simulink model "NavV1_0421_2021a"  (R2021a)
settings: Solver=FixedStepAuto  StartTime=0.0  StopTime=589  FixedStep=dt  RelTol=1e-3
values from neighbouring files (symbols this model uses):
  dt = 0.01    [initNavigation.m]
  g0 = 9.798    [initNavigation.m]
  GPSdt = 0.1    [initNavigation.m]
undefined symbols (not defined in the file or in its folder): DiscIntNeverNeededParam, magnitude, param
libraries: simulink x14, simulink_extras x11, sharedtransform x7, dspstat3 x4, aerolibtransform2 x2, dspsolvers x2, aerolibconvert2 x1
(part 2 of 3)

== system NavV1_0421_2021a/State estimation/Translation_estimate/V_Vertical_estimation ==
  note: Vd to Vh
  accel_Vertical_predict : Inport
  Sensor_data : Inport  Port=2
  Vertical_vaild_flag : Inport  Port=3
  Add : Sum
  Add1 : Sum  Inputs=++--
  Bus Selector : BusSelector  OutputSignals=QGC_sensor_reinit,TOF_Data.vH_TOF_m/s_TD,GPS_Data.vd_gps
  Bus Selector1 : BusSelector  OutputSignals=HTOF_vaild,HGPS_vaild
  Constant : Constant  Value=g0  OutDataTypeStr=single
  Delay : Delay  DelayLength=1  InitialConditionSource=Input port  ExternalReset=Level hold
      settings: InputPortMap=u0,r5,p4
  Gain : Gain  Gain=-1
  Gain2 : Gain  Gain=dt  SaturateOnIntegerOverflow=on  OutDataTypeStr=Inherit: Same as input  ParamDataTypeStr=Inherit: Same as input
  Scope : Scope
  Scope1 : Scope  NumInputPorts=3
  VH_correctionbyTOF : Subsystem
  VH_correctionbyTOF1 : Subsystem
  Vh_vertical_eastimate : Outport
  wires:
  Sensor_data/1 -> Bus Selector/1
  Bus Selector/3 -> VH_correctionbyTOF1/2(Vd_gps), Scope1/2, Delay/3  "<vd_gps>"
  Bus Selector/1 -> Delay/2  "<QGC_sensor_reinit>"
  accel_Vertical_predict/1 -> Scope/1, Add/1
  Constant/1 -> Add/2
  Add/1 -> Gain2/1
  Bus Selector/2 -> VH_correctionbyTOF/2(<vH_TOF_m/s_TD>), Scope1/3  "<vH_TOF_m/s_TD>"
  Add1/1 -> Scope1/1, Vh_vertical_eastimate/1, Delay/1, VH_correctionbyTOF/1(VH_k_1), VH_correctionbyTOF1/1(VH_k_1)
  Gain2/1 -> Gain/1
  VH_correctionbyTOF/1(VH_correctionbyTOF) -> Add1/3
  Delay/1 -> Add1/2
  Vertical_vaild_flag/1 -> Bus Selector1/1
  Bus Selector1/1 -> VH_correctionbyTOF/Enable  "<HTOF_vaild>"
  Bus Selector1/2 -> VH_correctionbyTOF1/Enable  "<HGPS_vaild>"
  VH_correctionbyTOF1/1(VH_correctionbyGPS) -> Add1/4
  Gain/1 -> Add1/1

== system NavV1_0421_2021a/State estimation/Translation_estimate/translate to N ==
  RotationData : Inport
  Sensor_data : Inport  Port=2
  Bus Selector2 : BusSelector  OutputSignals=IMU_Data.accl_B_m/s2_LPF
  Bus Selector3 : BusSelector  OutputSignals=DCM_b_n
  Product : Product  Multiplication=Matrix(*)
  Selector : Selector  InputPortWidth=3  IndexOptions=Index vector (dialog)  Indices=[1 2]  OutputSizes=1
  Selector1 : Selector  InputPortWidth=3  IndexOptions=Index vector (dialog)  Indices=[3]  OutputSizes=1
  accel_Horizontal_predict : Outport
  accel_Vertical_predict : Outport  Port=2
  wires:
  RotationData/1 -> Bus Selector3/1
  Bus Selector2/1 -> Product/2  "<accl_B_m/s2_LPF>"
  Bus Selector3/1 -> Product/1  "<DCM_b_n>"
  Sensor_data/1 -> Bus Selector2/1
  Product/1 -> Selector1/1, Selector/1
  Selector/1 -> accel_Horizontal_predict/1
  Selector1/1 -> accel_Vertical_predict/1

== system NavV1_0421_2021a/Sensor_Data_Process/GPS_Data_Process/LLA2NED/Subsystem1 ==
  QGC_sensor_reinit : Inport
  gps_LLA_rad : Inport  Port=2
  Detect Increase : simulink/Logic and Bit Operations/Detect Increase  vinit=0.0  OutDataTypeStr=boolean
  Switch : Switch  Criteria=u2 > Threshold
  Unit Delay : UnitDelay  SampleTime=-1  HasFrameUpgradeWarning=on
  init_gps_LLA0_rad : Outport
  wires:
  Unit Delay/1 -> Switch/3
  gps_LLA_rad/1 -> Switch/1
  Switch/1 -> init_gps_LLA0_rad/1, Unit Delay/1
  Detect Increase/1 -> Switch/2
  QGC_sensor_reinit/1 -> Detect Increase/1

== system NavV1_0421_2021a/State estimation/AHRS/AHRS Complementary filter/Complementary Filter ==
  fbxyz : Inport
  Fly_status : Inport  Port=2
  fb_estimatedValue : Inport  Port=3
  Cross-product : Subsystem
      mask DialogControl Control2 Prompt: Vector A×B
  Gain : Gain  Gain=GPS_accel_kp
  Gain2 : Gain  Gain=noGPS_accel_kp
  Gain3 : Gain  Gain=GPS_accel_ki*dt
  Gain4 : Gain  Gain=noGPS_accel_ki*dt
  Normalized : Subsystem
  Normalized1 : Subsystem
  Sum : Sum  Inputs=|++
  Sum1 : Sum  Inputs=|++
  Switch : Switch  Threshold=2
  w_bias : Outport
  wires:
  Normalized1/1(fb_estimatedValue_Normalized) -> Cross-product/2(vactor_B)
  Normalized/1(fb/g) -> Cross-product/1(vactor_A)
  fbxyz/1 -> Normalized/1(fb)
  fb_estimatedValue/1 -> Normalized1/1(fb_estimatedValue)
  Switch/1 -> w_bias/1
  Fly_status/1 -> Switch/2
  Sum/1 -> Switch/1
  Gain/1 -> Sum/1
  Gain3/1 -> Sum/2
  Cross-product/1(vactor_error_A&B) -> Gain4/1, Gain2/1, Gain3/1, Gain/1
  Gain2/1 -> Sum1/1
  Gain4/1 -> Sum1/2
  Sum1/1 -> Switch/3

== system NavV1_0421_2021a/State estimation/AHRS/AHRS Complementary filter/SmoothModel ==
  bias : Inport
  Demux : Demux  Outputs=3
  Moving Average : dspstat3/Moving Average  Method=Sliding window  ForgettingFactorPort=off  SpecifyWindowLength=on  WindowLength=10  ForgettingFactor=0.9  SimulateUsing=Code generation
  Moving Average1 : dspstat3/Moving Average  Method=Sliding window  ForgettingFactorPort=off  SpecifyWindowLength=on  WindowLength=10  ForgettingFactor=0.9  SimulateUsing=Code generation
  Moving Average2 : dspstat3/Moving Average  Method=Sliding window  ForgettingFactorPort=off  SpecifyWindowLength=on  WindowLength=10  ForgettingFactor=0.9  SimulateUsing=Code generation
  Mux : Mux  Inputs=3
  bias_smooth : Outport
  wires:
  Moving Average/1 -> Mux/1
  Moving Average1/1 -> Mux/2
  Demux/3 -> Moving Average2/1
  Demux/2 -> Moving Average1/1
  Moving Average2/1 -> Mux/3
  Demux/1 -> Moving Average/1
  bias/1 -> Demux/1
  Mux/1 -> bias_smooth/1  "gyro_B_rad/s_LPF"

== system NavV1_0421_2021a/State estimation/AHRS/AHRS Complementary filter/Subsystem6 ==
  m : Inport
  Add : Sum  Inputs=3
  Demux : Demux  Outputs=3
  Display : Display
  Display1 : Display
      settings: Decimation=3
  Divide : Product  Inputs=*/
  Dot Product : DotProduct  InputSameDT=on  OutDataTypeStr=Inherit: Inherit via internal rule
  Dot Product1 : DotProduct  InputSameDT=on  OutDataTypeStr=Inherit: Inherit via internal rule
  Dot Product2 : DotProduct  InputSameDT=on  OutDataTypeStr=Inherit: Inherit via internal rule
  Sqrt : Sqrt  SaturateOnIntegerOverflow=on
  m/|m| : Outport
  wires:
  Demux/2 -> Dot Product1/2, Dot Product1/1
  Demux/3 -> Dot Product2/2, Dot Product2/1
  Divide/1 -> Display1/1, m/|m|/1
  Add/1 -> Sqrt/1
  m/1 -> Demux/1, Divide/1
  Demux/1 -> Dot Product/1, Dot Product/2
  Dot Product1/1 -> Add/2
  Dot Product/1 -> Add/1
  Dot Product2/1 -> Add/3
  Sqrt/1 -> Display/1, Divide/2

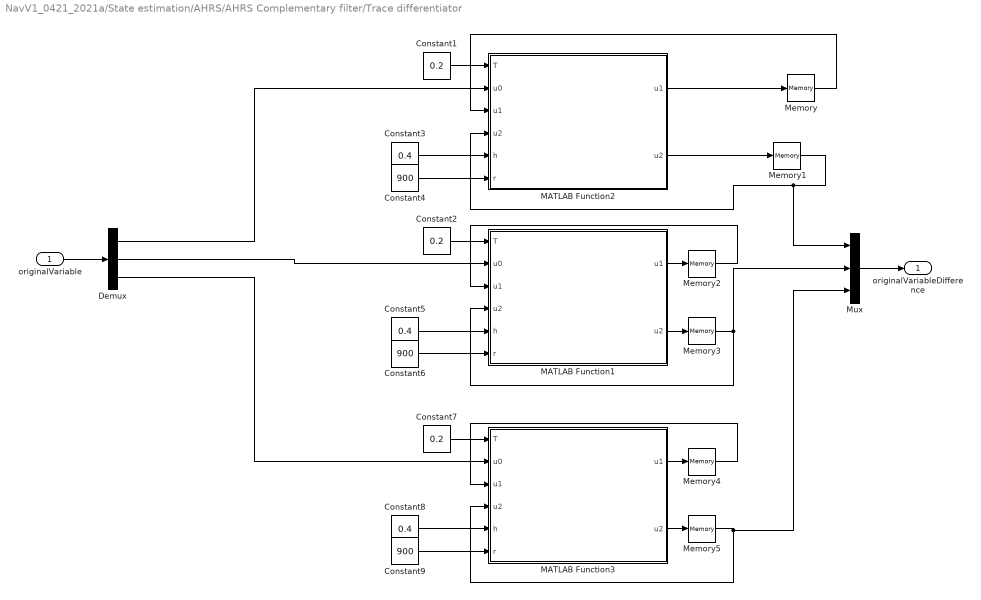
== system NavV1_0421_2021a/State estimation/AHRS/AHRS Complementary filter/Trace differentiator ==
  originalVariable : Inport
  Constant1 : Constant  Value=0.2  OutDataTypeStr=single
  Constant2 : Constant  Value=0.2  OutDataTypeStr=single
  Constant3 : Constant  Value=0.4  OutDataTypeStr=single
  Constant4 : Constant  Value=900  OutDataTypeStr=single
  Constant5 : Constant  Value=0.4  OutDataTypeStr=single
  Constant6 : Constant  Value=900  OutDataTypeStr=single
  Constant7 : Constant  Value=0.2  OutDataTypeStr=single
  Constant8 : Constant  Value=0.4  OutDataTypeStr=single
  Constant9 : Constant  Value=900  OutDataTypeStr=single
  Demux : Demux  Outputs=3
  MATLAB Function1 : MATLAB Function  TreatAsAtomicUnit=on
  MATLAB Function2 : MATLAB Function  TreatAsAtomicUnit=on
  MATLAB Function3 : MATLAB Function  TreatAsAtomicUnit=on
  Memory{,1..5} (6 alike) : Memory  InheritSampleTime=on
  Mux : Mux  Inputs=3
  originalVariableDifference : Outport
  wires:
  Demux/3 -> MATLAB Function3/2(u0)
  Demux/2 -> MATLAB Function1/2(u0)
  Demux/1 -> MATLAB Function2/2(u0)
  originalVariable/1 -> Demux/1
  Mux/1 -> originalVariableDifference/1
  Memory5/1 -> MATLAB Function3/4("u2 "), Mux/3
  Memory4/1 -> MATLAB Function3/3("u1 ")
  MATLAB Function3/2(u2) -> Memory5/1
  Constant8/1 -> MATLAB Function3/5(h)
  Constant7/1 -> MATLAB Function3/1(T)
  Constant9/1 -> MATLAB Function3/6(r)
  MATLAB Function3/1(u1) -> Memory4/1
  MATLAB Function1/1(u1) -> Memory2/1
  Constant6/1 -> MATLAB Function1/6(r)
  Constant2/1 -> MATLAB Function1/1(T)
  Constant5/1 -> MATLAB Function1/5(h)
  MATLAB Function1/2(u2) -> Memory3/1
  Memory2/1 -> MATLAB Function1/3("u1 ")
  Memory3/1 -> Mux/2, MATLAB Function1/4("u2 ")
  Memory1/1 -> MATLAB Function2/4("u2 "), Mux/1
  Memory/1 -> MATLAB Function2/3("u1 ")
  MATLAB Function2/2(u2) -> Memory1/1
  Constant3/1 -> MATLAB Function2/5(h)
  Constant1/1 -> MATLAB Function2/1(T)
  Constant4/1 -> MATLAB Function2/6(r)
  MATLAB Function2/1(u1) -> Memory/1

== system NavV1_0421_2021a/State estimation/AHRS/AHRS Complementary filter/UAV_accelerate_within_gravity_estimate ==
  Fly_status : Inport
  <DCM_b_n> : Inport  Port=2
  accel_GPS_ned : Inport  Port=3
  Add2 : Sum
  Constant : Constant  Value=[0;0;-1]
  Constant1 : Constant  Value=[0;0;0]  OutDataTypeStr=single
  Gain2 : Gain  Gain=g0
  Math Function1 : Math  Operator=transpose  SignedPower=on  SaturateOnIntegerOverflow=on
  Multiport Switch : MultiPortSwitch  Inputs=2  DataPortForDefault=Additional data port
  Product : Product  Multiplication=Matrix(*)  SaturateOnIntegerOverflow=on  OutDataTypeStr=Inherit: Same as first input
  Product1 : Product  Multiplication=Matrix(*)  SaturateOnIntegerOverflow=on  OutDataTypeStr=Inherit: Same as first input
  accelerate_within_gravity_estimate : Outport
  wires:
  <DCM_b_n>/1 -> Math Function1/1
  Math Function1/1 -> Product1/1, Product/1  "DCM_n_b"
  Product1/1 -> Add2/1
  accel_GPS_ned/1 -> Product1/2  "accel_GPS_ned"
  Product/1 -> Gain2/1
  Constant/1 -> Product/2
  Gain2/1 -> Multiport Switch/2, Add2/2
  Fly_status/1 -> Multiport Switch/1
  Multiport Switch/1 -> accelerate_within_gravity_estimate/1
  Add2/1 -> Multiport Switch/3
  Constant1/1 -> Multiport Switch/4

== system NavV1_0421_2021a/State estimation/AHRS/AHRS Complementary filter/chacheng6 ==
  In1 : Inport
  In2 : Inport  Port=2
  Bus Creator : BusCreator  Inputs=6
  Demux : Demux  Outputs=3
  Demux1 : Demux  Outputs=3
  Fcn : Fcn  Expr=u(2)*u(6)-u(3)*u(5)
  Fcn1 : Fcn  Expr=u(3)*u(4)-u(1)*u(6)
  Fcn2 : Fcn  Expr=u(1)*u(5)-u(2)*u(4)
  Mux2 : Mux  Inputs=3
  Out1 : Outport
  wires:
  Demux/1 -> Bus Creator/1
  Demux/2 -> Bus Creator/2
  Demux/3 -> Bus Creator/3
  Demux1/1 -> Bus Creator/4
  Demux1/2 -> Bus Creator/5
  Demux1/3 -> Bus Creator/6
  Bus Creator/1 -> Fcn/1, Fcn1/1, Fcn2/1
  Fcn/1 -> Mux2/1
  Fcn1/1 -> Mux2/2
  Fcn2/1 -> Mux2/3
  In1/1 -> Demux/1
  Mux2/1 -> Out1/1
  In2/1 -> Demux1/1

== system NavV1_0421_2021a/State estimation/AHRS/AHRS Complementary filter/manoeuvrable check ==
  note: 1：匀速运动或静止状态
      | 2：加速运动中
  accel_GPS_ned : Inport
  fbxyz1 : Inport  Port=2
  DCM_b_n : Inport  Port=3
  fixtype_GPS : Inport  Port=4
  Compare To Constant : simulink/Logic and Bit Operations/Compare To Constant  relop===  const=0  OutDataTypeStr=boolean
  Compare To Constant1 : simulink/Logic and Bit Operations/Compare To Constant  relop=>=  const=2  OutDataTypeStr=boolean
  Compare To Constant2 : simulink/Logic and Bit Operations/Compare To Constant  relop=>=  const=1  OutDataTypeStr=boolean
  Constant2 : Constant  OutDataTypeStr=uint8
  Constant3 : Constant  Value=2  OutDataTypeStr=uint8
  Logical Operator : Logic  AllPortsSameDT=off  OutDataTypeStr=boolean
  Logical Operator1 : Logic  Operator=OR  AllPortsSameDT=off  OutDataTypeStr=boolean
  Math Function : Math  Operator=magnitude^2  SaturateOnIntegerOverflow=on
  Product : Product  Multiplication=Matrix(*)
  Sqrt : Sqrt  SaturateOnIntegerOverflow=on
  Sum of Elements : Sum  Inputs=+
  Switch2 : Switch  Threshold=1
  manoeuvrable check : Subsystem
      mask DialogControl DescTextVar Prompt: manoeuvrable check
      mask DialogControl Control2 Prompt: flag = 0 : 机动状态
      mask DialogControl Control3 Prompt: flag = 1：静止/匀速状态
  Fly_status : Outport
  wires:
  accel_GPS_ned/1 -> Math Function/1
  Math Function/1 -> Sum of Elements/1
  fbxyz1/1 -> Product/2
  DCM_b_n/1 -> Product/1
  Product/1 -> manoeuvrable check/1(fn)
  manoeuvrable check/1(flag) -> Compare To Constant/1
  Sum of Elements/1 -> Sqrt/1
  Sqrt/1 -> Compare To Constant1/1
  Compare To Constant1/1 -> Logical Operator/2
  fixtype_GPS/1 -> Compare To Constant2/1
  Compare To Constant2/1 -> Logical Operator/1
  Compare To Constant/1 -> Logical Operator1/2
  Logical Operator/1 -> Logical Operator1/1
  Logical Operator1/1 -> Switch2/2
  Constant2/1 -> Switch2/3
  Constant3/1 -> Switch2/1
  Switch2/1 -> Fly_status/1

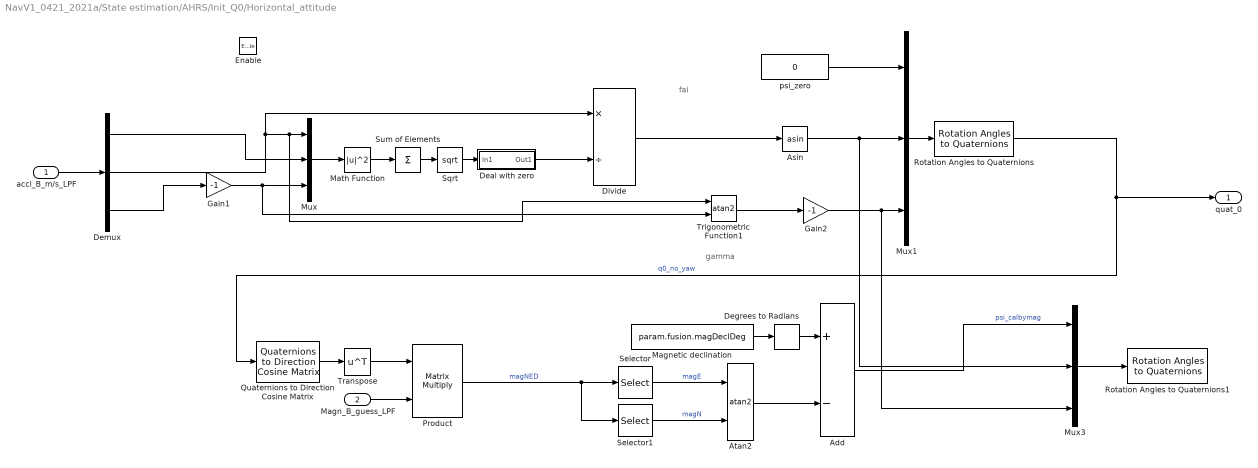
== system NavV1_0421_2021a/State estimation/AHRS/Init_Q0/Horizontal_attitude ==
  note: fai
  note: gamma
  accl_B_m/s_LPF : Inport  PortDimensions=3
  Magn_B_guess_LPF : Inport  Port=2
  Enable : EnablePort
  Add : Sum  Inputs=+-
  Asin : Trigonometry  Operator=asin
  Atan2 : Trigonometry  Operator=atan2
  Deal with zero : Subsystem
  Degrees to Radians : simulink_extras/Transformations/Degrees to Radians
  Demux : Demux  Outputs=3
  Divide : Product  Inputs=*/  OutDataTypeStr=single
  Gain1 : Gain  Gain=-1
  Gain2 : Gain  Gain=-1
  Magnetic declination : Constant  Value=param.fusion.magDeclDeg  OutDataTypeStr=single
  Math Function : Math  Operator=magnitude^2  SaturateOnIntegerOverflow=on
  Mux : Mux  Inputs=3
  Mux1 : Mux  Inputs=3
  Mux3 : Mux  Inputs=3
  Product : Product  Multiplication=Matrix(*)
  Quaternions to Direction Cosine Matrix : sharedtransform/Quaternions to  Direction Cosine Matrix  aMode=aMode
      settings: SourceProductBaseCode=AE,PW,DR,MT,UV,VE
  Rotation Angles to Quaternions : sharedtransform/Rotation Angles to Quaternions  rotationOrder=ZYX  aMode=aMode
      settings: SourceProductBaseCode=AE,PW,DR,MT,UV,VE
  Rotation Angles to Quaternions1 : sharedtransform/Rotation Angles to Quaternions  rotationOrder=ZYX  aMode=aMode
      settings: SourceProductBaseCode=AE,PW,DR,MT,UV,VE
  Selector : Selector  InputPortWidth=3  IndexOptions=Index vector (dialog)  Indices=[2]  OutputSizes=1
  Selector1 : Selector  InputPortWidth=3  IndexOptions=Index vector (dialog)  Indices=[1]  OutputSizes=1
  Sqrt : Sqrt  SaturateOnIntegerOverflow=on
  Sum of Elements : Sum  Inputs=+
  Transpose : Math  Operator=transpose  SaturateOnIntegerOverflow=on
  Trigonometric Function1 : Trigonometry  Operator=atan2
  psi_zero : Constant  Value=0  OutDataTypeStr=single
  quat_0 : Outport  PortDimensions=4
  wires:
  accl_B_m/s_LPF/1 -> Demux/1
  Sqrt/1 -> Deal with zero/1(In1)
  Deal with zero/1(Out1) -> Divide/2
  Trigonometric Function1/1 -> Gain2/1
  Demux/1 -> Mux/2
  Demux/2 -> Trigonometric Function1/1, Mux/1, Divide/1
  Demux/3 -> Gain1/1
  Sum of Elements/1 -> Sqrt/1
  Divide/1 -> Asin/1
  Mux/1 -> Math Function/1
  Math Function/1 -> Sum of Elements/1
  Mux1/1 -> Rotation Angles to Quaternions/1
  psi_zero/1 -> Mux1/1
  Asin/1 -> Mux3/2, Mux1/2
  Gain2/1 -> Mux3/3, Mux1/3
  Rotation Angles to Quaternions/1 -> quat_0/1, Quaternions to Direction Cosine Matrix/1  "q0_no_yaw"
  Quaternions to Direction Cosine Matrix/1 -> Transpose/1
  Magn_B_guess_LPF/1 -> Product/2
  Product/1 -> Selector/1, Selector1/1  "magNED"
  Selector1/1 -> Atan2/2  "magN"
  Selector/1 -> Atan2/1  "magE"
  Atan2/1 -> Add/2
  Magnetic declination/1 -> Degrees to Radians/1
  Degrees to Radians/1 -> Add/1
  Add/1 -> Mux3/1  "psi_calbymag"
  Mux3/1 -> Rotation Angles to Quaternions1/1
  Transpose/1 -> Product/1
  Gain1/1 -> Trigonometric Function1/2, Mux/3

== system NavV1_0421_2021a/State estimation/AHRS/att_update/uniformization ==
  Q i : Inport  PortDimensions=4
  Constant : Constant  Value=1e-20
  Dot Product1 : DotProduct  InputSameDT=on  OutDataTypeStr=Inherit: Inherit via internal rule
  Math Function : Math  Operator=sqrt  SignedPower=on  SaturateOnIntegerOverflow=on
  Product : Product  Inputs=*/  SaturateOnIntegerOverflow=on  OutDataTypeStr=Inherit: Same as first input
  Sum : Sum  Inputs=|++  SaturateOnIntegerOverflow=on
  Q o : Outport
  wires:
  Q i/1 -> Dot Product1/2, Dot Product1/1, Product/1
  Dot Product1/1 -> Math Function/1
  Math Function/1 -> Sum/1
  Product/1 -> Q o/1
  Constant/1 -> Sum/2
  Sum/1 -> Product/2

== system NavV1_0421_2021a/State estimation/Translation_estimate/Rxy_Horizontal_estimation/Integrator_R_Horizontal ==
  Vn : Inport
  dR : Inport  Port=2
  Sensor_data2 : Inport  Port=3
  Bus Selector : BusSelector  OutputSignals=QGC_sensor_reinit,GPS_Data.pos_N_gps,GPS_Data.pos_E_gps
  Delay : Delay  DelayLength=1  InitialConditionSource=Input port  ExternalReset=Level hold
      settings: InputPortMap=u0,r5,p4
  Gain : Gain  Gain=0.8
  Gain2 : Gain  Gain=dt  SaturateOnIntegerOverflow=on  OutDataTypeStr=Inherit: Same as input  ParamDataTypeStr=Inherit: Same as input
  Mux : Mux  Inputs=2
  Sum : Sum  Inputs=|++-
  R_n&e : Outport
  wires:
  Delay/1 -> Sum/2
  Mux/1 -> Delay/3
  Bus Selector/3 -> Mux/2  "<pos_E_gps>"
  Bus Selector/2 -> Mux/1  "<pos_N_gps>"
  Bus Selector/1 -> Delay/2  "<QGC_sensor_reinit>"
  Sensor_data2/1 -> Bus Selector/1
  Sum/1 -> Delay/1, R_n&e/1
  Gain2/1 -> Sum/1
  Vn/1 -> Gain2/1
  dR/1 -> Gain/1
  Gain/1 -> Sum/3

== system NavV1_0421_2021a/State estimation/Translation_estimate/Rxy_Horizontal_estimation/Rxy_kalman filter2 ==
  X : Inport
  Z : Inport  Port=2
  Enable : Inport  Port=3
  Constant : Constant  Value=F  OutDataTypeStr=single
  Constant1 : Constant  Value=Q  OutDataTypeStr=single
  Constant2 : Constant  Value=R  OutDataTypeStr=single
  Constant3 : Constant  Value=P0  OutDataTypeStr=single
  Constant4 : Constant  Value=H  OutDataTypeStr=single
  Vxy kalman filter : Subsystem  TreatAsAtomicUnit=on
  XOut : Outport
  wires:
  X/1 -> Vxy kalman filter/7(X)
  Constant/1 -> Vxy kalman filter/2(F), Vxy kalman filter/3(G)
  Z/1 -> Vxy kalman filter/1(Z)
  Constant3/1 -> Vxy kalman filter/8(P0)
  Constant2/1 -> Vxy kalman filter/6(R)
  Constant4/1 -> Vxy kalman filter/4(H)
  Constant1/1 -> Vxy kalman filter/5(Q)
  Vxy kalman filter/1(XOut) -> XOut/1
  Enable/1 -> Vxy kalman filter/9(Enable)

== system NavV1_0421_2021a/State estimation/Translation_estimate/Subsystem/VH_correctionbyTOF ==
  H_k_1 : Inport
  <H_TOF_m/s_TD> : Inport  Port=2
  Enable : EnablePort
  Add1 : Sum  Inputs=+-
  Gain : Gain  Gain=0.95
  Memory1 : Memory
  H_correctionbyTOF : Outport
  wires:
  Gain/1 -> H_correctionbyTOF/1
  Add1/1 -> Gain/1
  <H_TOF_m/s_TD>/1 -> Add1/2
  H_k_1/1 -> Memory1/1
  Memory1/1 -> Add1/1

== system NavV1_0421_2021a/State estimation/Translation_estimate/Subsystem/VH_correctionbyTOF1 ==
  H_k_1 : Inport
  H_gps : Inport  Port=2
  Enable : EnablePort
  Add1 : Sum  Inputs=+-
  Gain : Gain  Gain=0.8
  Memory1 : Memory
  H_correctionbyGPS : Outport
  wires:
  H_k_1/1 -> Memory1/1
  H_gps/1 -> Add1/2
  Add1/1 -> Gain/1
  Gain/1 -> H_correctionbyGPS/1
  Memory1/1 -> Add1/1

== system NavV1_0421_2021a/State estimation/Translation_estimate/V_Horizontal_estimation/Integrator_V_Horizontal ==
  An : Inport
  dv : Inport  Port=2
  Sensor_data2 : Inport  Port=3
  Bus Selector : BusSelector  OutputSignals=QGC_sensor_reinit,GPS_Data.vn_gps,GPS_Data.ve_gps
  Delay : Delay  DelayLength=1  InitialConditionSource=Input port  ExternalReset=Level hold
      settings: InputPortMap=u0,r5,p4
  Gain : Gain
  Gain2 : Gain  Gain=dt  SaturateOnIntegerOverflow=on  OutDataTypeStr=Inherit: Same as input  ParamDataTypeStr=Inherit: Same as input
  Mux : Mux  Inputs=2
  Sum : Sum  Inputs=|++-
  V_n&e : Outport
  wires:
  An/1 -> Gain2/1
  Gain2/1 -> Sum/1
  Sum/1 -> V_n&e/1, Delay/1
  Sensor_data2/1 -> Bus Selector/1
  Bus Selector/1 -> Delay/2  "<QGC_sensor_reinit>"
  Bus Selector/2 -> Mux/1  "<vn_gps>"
  Bus Selector/3 -> Mux/2  "<ve_gps>"
  Mux/1 -> Delay/3
  Delay/1 -> Sum/2
  dv/1 -> Gain/1
  Gain/1 -> Sum/3

== system NavV1_0421_2021a/State estimation/Translation_estimate/V_Horizontal_estimation/Rxy_kalman filter1 ==
  X : Inport
  Z : Inport  Port=2
  Enable : Inport  Port=3
  Constant : Constant  Value=F  OutDataTypeStr=single
  Constant1 : Constant  Value=Q  OutDataTypeStr=single
  Constant2 : Constant  Value=R  OutDataTypeStr=single
  Constant3 : Constant  Value=P0  OutDataTypeStr=single
  Constant4 : Constant  Value=H  OutDataTypeStr=single
  Vxy kalman filter : Subsystem  TreatAsAtomicUnit=on
  XOut : Outport
  wires:
  Enable/1 -> Vxy kalman filter/9(Enable)
  Vxy kalman filter/1(XOut) -> XOut/1
  Constant1/1 -> Vxy kalman filter/5(Q)
  Constant4/1 -> Vxy kalman filter/4(H)
  Constant2/1 -> Vxy kalman filter/6(R)
  Constant3/1 -> Vxy kalman filter/8(P0)
  Z/1 -> Vxy kalman filter/1(Z)
  Constant/1 -> Vxy kalman filter/3(G), Vxy kalman filter/2(F)
  X/1 -> Vxy kalman filter/7(X)

== system NavV1_0421_2021a/State estimation/Translation_estimate/V_Vertical_estimation/VH_correctionbyTOF ==
  VH_k_1 : Inport
  <vH_TOF_m/s_TD> : Inport  Port=2
  Enable : EnablePort
  Add1 : Sum  Inputs=+-
  Gain : Gain  Gain=0.95
  Memory1 : Memory
  VH_correctionbyTOF : Outport
  wires:
  Gain/1 -> VH_correctionbyTOF/1
  Add1/1 -> Gain/1
  <vH_TOF_m/s_TD>/1 -> Add1/2
  VH_k_1/1 -> Memory1/1
  Memory1/1 -> Add1/1

== system NavV1_0421_2021a/State estimation/Translation_estimate/V_Vertical_estimation/VH_correctionbyTOF1 ==
  VH_k_1 : Inport
  Vd_gps : Inport  Port=2
  Enable : EnablePort
  Add1 : Sum  Inputs=+-
  Gain : Gain  Gain=0.8
  Memory1 : Memory
  VH_correctionbyGPS : Outport
  wires:
  VH_k_1/1 -> Memory1/1
  Vd_gps/1 -> Add1/2
  Add1/1 -> Gain/1
  Gain/1 -> VH_correctionbyGPS/1
  Memory1/1 -> Add1/1

== system NavV1_0421_2021a/State estimation/AHRS/AHRS Complementary filter/Complementary Filter/Cross-product ==
  vactor_A : Inport
  vactor_B : Inport  Port=2
  Bus Creator : BusCreator  Inputs=6
  Demux : Demux  Outputs=3
  Demux1 : Demux  Outputs=3
  Fcn : Fcn  Expr=u(2)*u(6)-u(3)*u(5)
  Fcn1 : Fcn  Expr=u(3)*u(4)-u(1)*u(6)
  Fcn2 : Fcn  Expr=u(1)*u(5)-u(2)*u(4)
  Mux2 : Mux  Inputs=3
  vactor_error_A&B : Outport
  wires:
  vactor_B/1 -> Demux1/1
  Mux2/1 -> vactor_error_A&B/1
  vactor_A/1 -> Demux/1
  Fcn2/1 -> Mux2/3
  Fcn1/1 -> Mux2/2
  Fcn/1 -> Mux2/1
  Bus Creator/1 -> Fcn/1, Fcn1/1, Fcn2/1
  Demux1/3 -> Bus Creator/6
  Demux1/2 -> Bus Creator/5
  Demux1/1 -> Bus Creator/4
  Demux/3 -> Bus Creator/3
  Demux/2 -> Bus Creator/2
  Demux/1 -> Bus Creator/1

== system NavV1_0421_2021a/State estimation/AHRS/AHRS Complementary filter/Complementary Filter/Normalized ==
  fb : Inport
  Divide : Product  Inputs=*/
  Math Function : Math  Operator=magnitude^2  SaturateOnIntegerOverflow=on
  Sqrt : Sqrt  SaturateOnIntegerOverflow=on
  Sum of Elements : Sum  Inputs=+
  fb/g : Outport
  wires:
  Sqrt/1 -> Divide/2
  fb/1 -> Math Function/1, Divide/1
  Sum of Elements/1 -> Sqrt/1
  Divide/1 -> fb/g/1
  Math Function/1 -> Sum of Elements/1

== system NavV1_0421_2021a/State estimation/AHRS/AHRS Complementary filter/Complementary Filter/Normalized1 ==
  fb_estimatedValue : Inport
  Divide : Product  Inputs=*/
  Math Function : Math  Operator=magnitude^2  SaturateOnIntegerOverflow=on
  Sqrt : Sqrt  SaturateOnIntegerOverflow=on
  Sum of Elements : Sum  Inputs=+
  fb_estimatedValue_Normalized : Outport
  wires:
  Sqrt/1 -> Divide/2
  fb_estimatedValue/1 -> Math Function/1, Divide/1
  Sum of Elements/1 -> Sqrt/1
  Divide/1 -> fb_estimatedValue_Normalized/1
  Math Function/1 -> Sum of Elements/1

== system NavV1_0421_2021a/State estimation/AHRS/AHRS Complementary filter/manoeuvrable check/manoeuvrable check ==
  fn : Inport
  manoeuvrable check : MATLAB Function  TreatAsAtomicUnit=on
  flag : Outport
  wires:
  fn/1 -> manoeuvrable check/1(fn)
  manoeuvrable check/1(flag) -> flag/1

== system NavV1_0421_2021a/State estimation/AHRS/Init_Q0/Horizontal_attitude/Deal with zero ==
  In1 : Inport
  Add5 : Sum
  Constant1 : Constant  Value=1e-6  OutDataTypeStr=single
  Out1 : Outport
  wires:
  Add5/1 -> Out1/1
  In1/1 -> Add5/1
  Constant1/1 -> Add5/2

== system NavV1_0421_2021a/State estimation/Translation_estimate/Rxy_Horizontal_estimation/Rxy_kalman filter2/Vxy kalman filter ==
  Z : Inport
  F : Inport  Port=2
  G : Inport  Port=3
  H : Inport  Port=4
  Q : Inport  Port=5
  R : Inport  Port=6
  X : Inport  Port=7
  P0 : Inport  Port=8
  Enable : Inport  Port=9
  Add1 : Sum
  Delay : Delay  DelayLength=1  InitialConditionSource=Input port
      settings: InputPortMap=u0,p4
  Gain4 : Gain  Gain=0.5
  Math Function : Math  Operator=transpose  SignedPower=on  SaturateOnIntegerOverflow=on
  kalman : Subsystem
  XOut : Outport
  wires:
  Enable/1 -> kalman/9(Enable)
  kalman/2(XOut) -> XOut/1
  kalman/1(POut) -> Add1/1, Math Function/1
  X/1 -> kalman/8(X)
  R/1 -> kalman/6(R)
  Q/1 -> kalman/5(Q)
  H/1 -> kalman/4(H)
  G/1 -> kalman/3(G)
  F/1 -> kalman/2(F)
  Z/1 -> kalman/1(Z)
  Math Function/1 -> Add1/2
  Add1/1 -> Gain4/1
  Delay/1 -> kalman/7(P)
  Gain4/1 -> Delay/1
  P0/1 -> Delay/2

== system NavV1_0421_2021a/State estimation/Translation_estimate/V_Horizontal_estimation/Rxy_kalman filter1/Vxy kalman filter ==
  Z : Inport
  F : Inport  Port=2
  G : Inport  Port=3
  H : Inport  Port=4
  Q : Inport  Port=5
  R : Inport  Port=6
  X : Inport  Port=7
  P0 : Inport  Port=8
  Enable : Inport  Port=9
  Add1 : Sum
  Delay : Delay  DelayLength=1  InitialConditionSource=Input port
      settings: InputPortMap=u0,p4
  Gain4 : Gain  Gain=0.5
  Math Function : Math  Operator=transpose  SignedPower=on  SaturateOnIntegerOverflow=on
  kalman : Subsystem
  XOut : Outport
  wires:
  P0/1 -> Delay/2
  Gain4/1 -> Delay/1
  Delay/1 -> kalman/7(P)
  Add1/1 -> Gain4/1
  Math Function/1 -> Add1/2
  Z/1 -> kalman/1(Z)
  F/1 -> kalman/2(F)
  G/1 -> kalman/3(G)
  H/1 -> kalman/4(H)
  Q/1 -> kalman/5(Q)
  R/1 -> kalman/6(R)
  X/1 -> kalman/8(X)
  kalman/1(POut) -> Math Function/1, Add1/1
  kalman/2(XOut) -> XOut/1
  Enable/1 -> kalman/9(Enable)

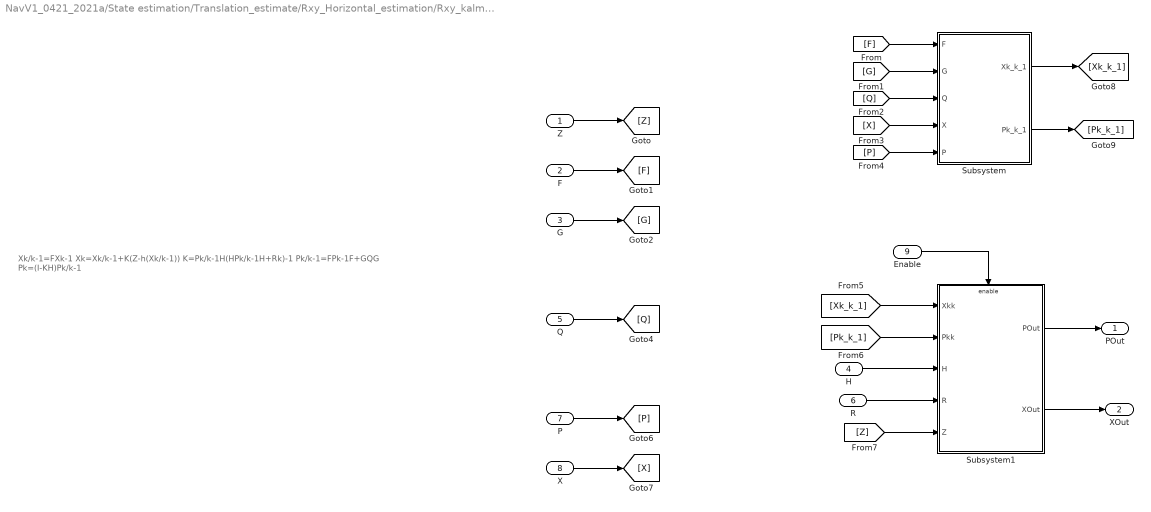
== system NavV1_0421_2021a/State estimation/Translation_estimate/Rxy_Horizontal_estimation/Rxy_kalman filter2/Vxy kalman filter/kalman ==
  note: Xk/k-1=FXk-1
      | Xk=Xk/k-1+K(Z-h(Xk/k-1))
      | K=Pk/k-1H(HPk/k-1H+Rk)-1
      | Pk/k-1=FPk-1F+GQG
      | Pk=(I-KH)Pk/k-1
  Z : Inport
  F : Inport  Port=2
  G : Inport  Port=3
  H : Inport  Port=4
  Q : Inport  Port=5
  R : Inport  Port=6
  P : Inport  Port=7
  X : Inport  Port=8
  Enable : Inport  Port=9
  Subsystem : Subsystem
  Subsystem1 : Subsystem
  POut : Outport
  XOut : Outport  Port=2
  wires:
  [Z] -> Subsystem1/5(Z)
  Enable/1 -> Subsystem1/Enable
  [Pk_k_1] -> Subsystem1/2(Pkk)
  [Xk_k_1] -> Subsystem1/1(Xkk)
  Subsystem1/2(XOut) -> XOut/1
  Subsystem1/1(POut) -> POut/1
  R/1 -> Subsystem1/4(R)
  H/1 -> Subsystem1/3(H)
  Subsystem/2(Pk_k_1) -> [Pk_k_1]
  Subsystem/1(Xk_k_1) -> [Xk_k_1]
  [P] -> Subsystem/5(P)
  [X] -> Subsystem/4(X)
  [Q] -> Subsystem/3(Q)
  [G] -> Subsystem/2(G)
  [F] -> Subsystem/1(F)
  Z/1 -> [Z]
  F/1 -> [F]
  G/1 -> [G]
  Q/1 -> [Q]
  P/1 -> [P]
  X/1 -> [X]

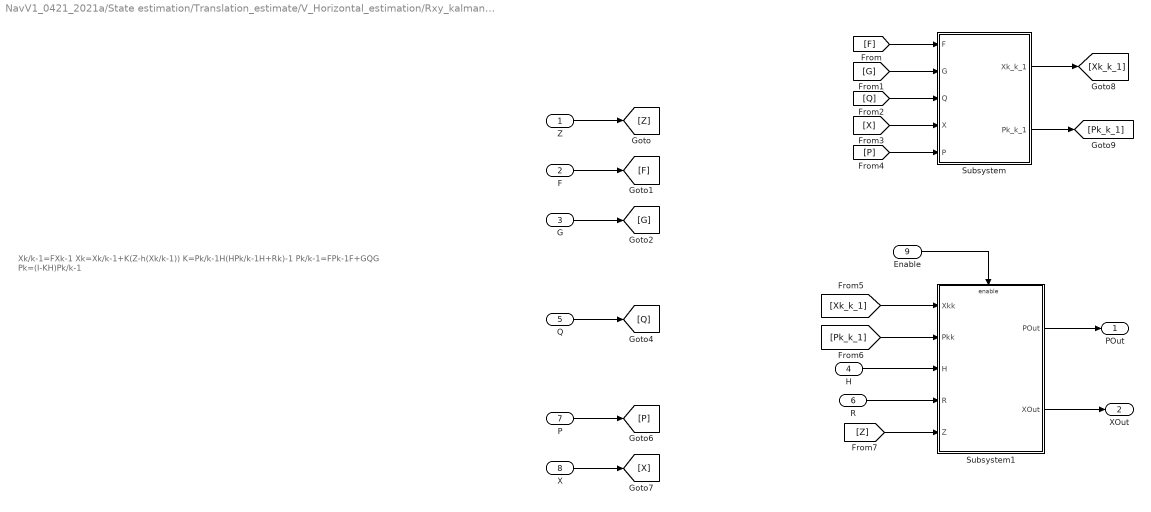
== system NavV1_0421_2021a/State estimation/Translation_estimate/V_Horizontal_estimation/Rxy_kalman filter1/Vxy kalman filter/kalman ==
  note: Xk/k-1=FXk-1
      | Xk=Xk/k-1+K(Z-h(Xk/k-1))
      | K=Pk/k-1H(HPk/k-1H+Rk)-1
      | Pk/k-1=FPk-1F+GQG
      | Pk=(I-KH)Pk/k-1
  Z : Inport
  F : Inport  Port=2
  G : Inport  Port=3
  H : Inport  Port=4
  Q : Inport  Port=5
  R : Inport  Port=6
  P : Inport  Port=7
  X : Inport  Port=8
  Enable : Inport  Port=9
  Subsystem : Subsystem
  Subsystem1 : Subsystem
  POut : Outport
  XOut : Outport  Port=2
  wires:
  X/1 -> [X]
  P/1 -> [P]
  Q/1 -> [Q]
  G/1 -> [G]
  F/1 -> [F]
  Z/1 -> [Z]
  [F] -> Subsystem/1(F)
  [G] -> Subsystem/2(G)
  [Q] -> Subsystem/3(Q)
  [X] -> Subsystem/4(X)
  [P] -> Subsystem/5(P)
  Subsystem/1(Xk_k_1) -> [Xk_k_1]
  Subsystem/2(Pk_k_1) -> [Pk_k_1]
  H/1 -> Subsystem1/3(H)
  R/1 -> Subsystem1/4(R)
  Subsystem1/1(POut) -> POut/1
  Subsystem1/2(XOut) -> XOut/1
  [Xk_k_1] -> Subsystem1/1(Xkk)
  [Pk_k_1] -> Subsystem1/2(Pkk)
  Enable/1 -> Subsystem1/Enable
  [Z] -> Subsystem1/5(Z)

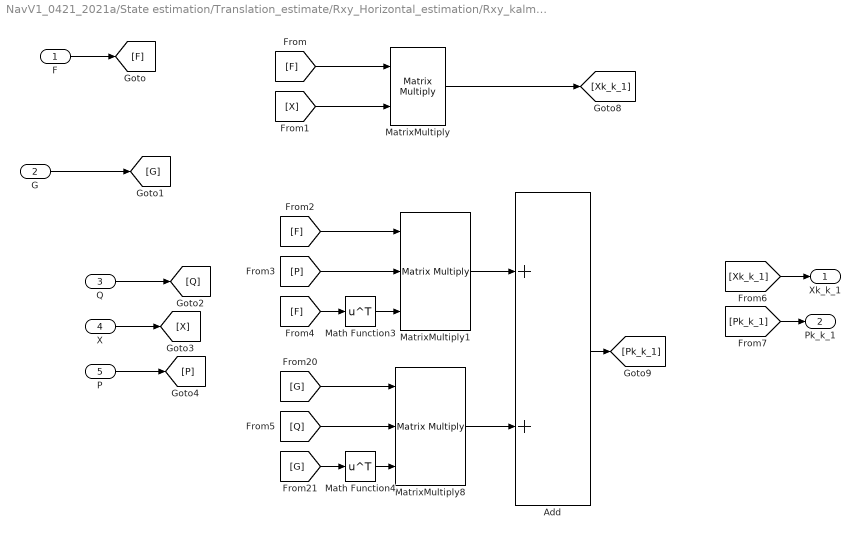
== system NavV1_0421_2021a/State estimation/Translation_estimate/Rxy_Horizontal_estimation/Rxy_kalman filter2/Vxy kalman filter/kalman/Subsystem ==
  F : Inport
  G : Inport  Port=2
  Q : Inport  Port=3
  X : Inport  Port=4
  P : Inport  Port=5
  Add : Sum
  Math Function3 : Math  Operator=transpose  SignedPower=on  SaturateOnIntegerOverflow=on
  Math Function4 : Math  Operator=transpose  SignedPower=on  SaturateOnIntegerOverflow=on
  MatrixMultiply : Product  Multiplication=Matrix(*)
  MatrixMultiply1 : Product  Inputs=3  Multiplication=Matrix(*)
  MatrixMultiply8 : Product  Inputs=3  Multiplication=Matrix(*)
  Xk_k_1 : Outport
  Pk_k_1 : Outport  Port=2
  wires:
  [Pk_k_1] -> Pk_k_1/1
  [Xk_k_1] -> Xk_k_1/1
  P/1 -> [P]
  X/1 -> [X]
  Q/1 -> [Q]
  G/1 -> [G]
  F/1 -> [F]
  [F] -> MatrixMultiply/1
  [G] -> Math Function4/1
  [X] -> MatrixMultiply/2
  MatrixMultiply8/1 -> Add/2
  [G] -> MatrixMultiply8/1
  Add/1 -> [Pk_k_1]
  [F] -> MatrixMultiply1/1
  [P] -> MatrixMultiply1/2
  Math Function3/1 -> MatrixMultiply1/3
  [F] -> Math Function3/1
  MatrixMultiply1/1 -> Add/1
  MatrixMultiply/1 -> [Xk_k_1]
  [Q] -> MatrixMultiply8/2
  Math Function4/1 -> MatrixMultiply8/3

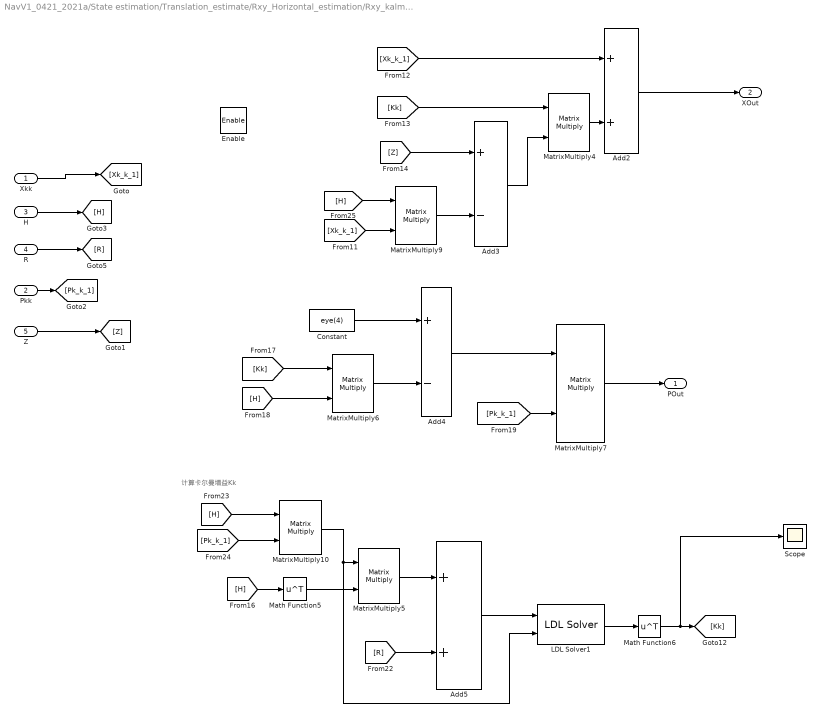
== system NavV1_0421_2021a/State estimation/Translation_estimate/Rxy_Horizontal_estimation/Rxy_kalman filter2/Vxy kalman filter/kalman/Subsystem1 ==
  note: 计算卡尔曼增益Kk
  Xkk : Inport
  Pkk : Inport  Port=2
  H : Inport  Port=3
  R : Inport  Port=4
  Z : Inport  Port=5
  Enable : EnablePort
  Add2 : Sum
  Add3 : Sum  Inputs=+-
  Add4 : Sum  Inputs=+-
  Add5 : Sum
  Constant : Constant  Value=eye(4)  OutDataTypeStr=single
  LDL Solver1 : dspsolvers/LDL Solver  errmode=Warning
      settings: SourceProductBaseCode=DS  RTWMemSecFuncInitTerm=Default  RTWMemSecFuncExecute=Default  RTWMemSecDataConstants=Default  RTWMemSecDataInternal=Default  RTWMemSecDataParameters=Default
  Math Function5 : Math  Operator=transpose  SignedPower=on  SaturateOnIntegerOverflow=on
  Math Function6 : Math  Operator=transpose  SignedPower=on  SaturateOnIntegerOverflow=on
  MatrixMultiply{4..7,9..10} (6 alike) : Product  Multiplication=Matrix(*)
  Scope : Scope
  POut : Outport
  XOut : Outport  Port=2
  wires:
  Pkk/1 -> [Pk_k_1]
  Z/1 -> [Z]
  Xkk/1 -> [Xk_k_1]
  Add2/1 -> XOut/1
  H/1 -> [H]
  MatrixMultiply6/1 -> Add4/2
  Add5/1 -> LDL Solver1/1
  R/1 -> [R]
  [Pk_k_1] -> MatrixMultiply7/2
  [Xk_k_1] -> MatrixMultiply9/2
  [H] -> MatrixMultiply9/1
  [H] -> MatrixMultiply6/2
  [Xk_k_1] -> Add2/1
  [Kk] -> MatrixMultiply6/1
  Constant/1 -> Add4/1
  [R] -> Add5/2
  [Pk_k_1] -> MatrixMultiply10/2
  [H] -> Math Function5/1
  LDL Solver1/1 -> Math Function6/1
  MatrixMultiply5/1 -> Add5/1
  MatrixMultiply10/1 -> LDL Solver1/2, MatrixMultiply5/1
  [Z] -> Add3/1
  [Kk] -> MatrixMultiply4/1
  MatrixMultiply4/1 -> Add2/2
  Add4/1 -> MatrixMultiply7/1
  Math Function6/1 -> [Kk], Scope/1
  Math Function5/1 -> MatrixMultiply5/2
  Add3/1 -> MatrixMultiply4/2
  [H] -> MatrixMultiply10/1
  MatrixMultiply7/1 -> POut/1
  MatrixMultiply9/1 -> Add3/2

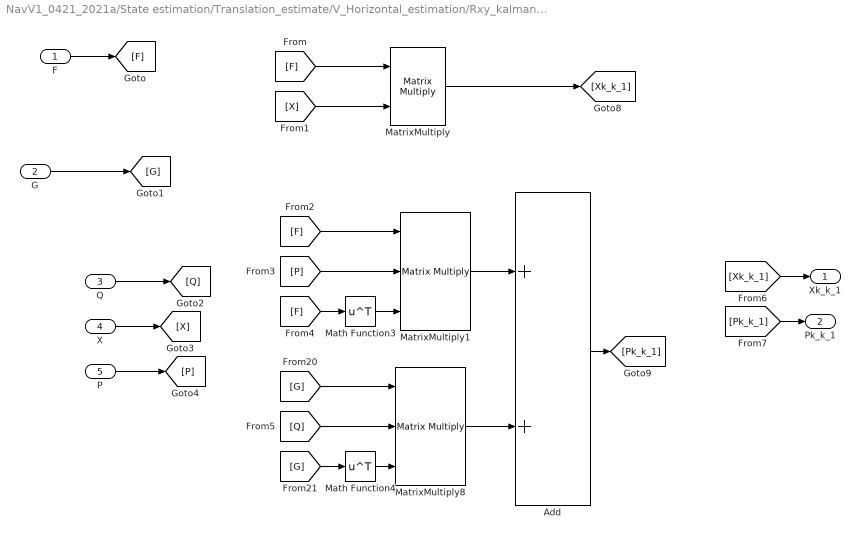
== system NavV1_0421_2021a/State estimation/Translation_estimate/V_Horizontal_estimation/Rxy_kalman filter1/Vxy kalman filter/kalman/Subsystem ==
  F : Inport
  G : Inport  Port=2
  Q : Inport  Port=3
  X : Inport  Port=4
  P : Inport  Port=5
  Add : Sum
  Math Function3 : Math  Operator=transpose  SignedPower=on  SaturateOnIntegerOverflow=on
  Math Function4 : Math  Operator=transpose  SignedPower=on  SaturateOnIntegerOverflow=on
  MatrixMultiply : Product  Multiplication=Matrix(*)
  MatrixMultiply1 : Product  Inputs=3  Multiplication=Matrix(*)
  MatrixMultiply8 : Product  Inputs=3  Multiplication=Matrix(*)
  Xk_k_1 : Outport
  Pk_k_1 : Outport  Port=2
  wires:
  Math Function4/1 -> MatrixMultiply8/3
  [Q] -> MatrixMultiply8/2
  MatrixMultiply/1 -> [Xk_k_1]
  MatrixMultiply1/1 -> Add/1
  [F] -> Math Function3/1
  Math Function3/1 -> MatrixMultiply1/3
  [P] -> MatrixMultiply1/2
  [F] -> MatrixMultiply1/1
  Add/1 -> [Pk_k_1]
  [G] -> MatrixMultiply8/1
  MatrixMultiply8/1 -> Add/2
  [X] -> MatrixMultiply/2
  [G] -> Math Function4/1
  [F] -> MatrixMultiply/1
  F/1 -> [F]
  G/1 -> [G]
  Q/1 -> [Q]
  X/1 -> [X]
  P/1 -> [P]
  [Xk_k_1] -> Xk_k_1/1
  [Pk_k_1] -> Pk_k_1/1

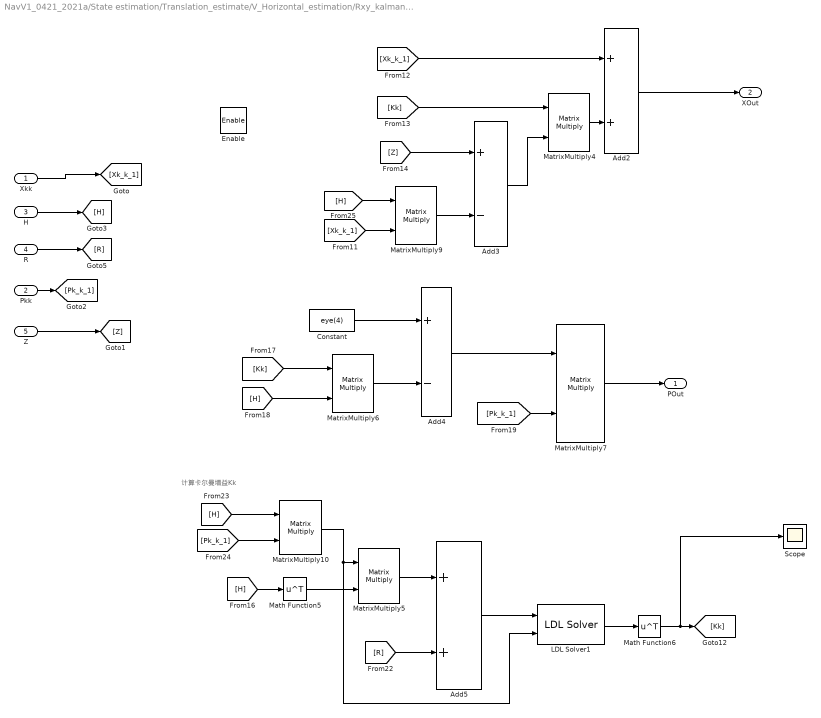
== system NavV1_0421_2021a/State estimation/Translation_estimate/V_Horizontal_estimation/Rxy_kalman filter1/Vxy kalman filter/kalman/Subsystem1 ==
  note: 计算卡尔曼增益Kk
  Xkk : Inport
  Pkk : Inport  Port=2
  H : Inport  Port=3
  R : Inport  Port=4
  Z : Inport  Port=5
  Enable : EnablePort
  Add2 : Sum
  Add3 : Sum  Inputs=+-
  Add4 : Sum  Inputs=+-
  Add5 : Sum
  Constant : Constant  Value=eye(4)  OutDataTypeStr=single
  LDL Solver1 : dspsolvers/LDL Solver  errmode=Warning
      settings: SourceProductBaseCode=DS  RTWMemSecFuncInitTerm=Default  RTWMemSecFuncExecute=Default  RTWMemSecDataConstants=Default  RTWMemSecDataInternal=Default  RTWMemSecDataParameters=Default
  Math Function5 : Math  Operator=transpose  SignedPower=on  SaturateOnIntegerOverflow=on
  Math Function6 : Math  Operator=transpose  SignedPower=on  SaturateOnIntegerOverflow=on
  MatrixMultiply{4..7,9..10} (6 alike) : Product  Multiplication=Matrix(*)
  Scope : Scope
  POut : Outport
  XOut : Outport  Port=2
  wires:
  MatrixMultiply9/1 -> Add3/2
  MatrixMultiply7/1 -> POut/1
  [H] -> MatrixMultiply10/1
  Add3/1 -> MatrixMultiply4/2
  Math Function5/1 -> MatrixMultiply5/2
  Math Function6/1 -> Scope/1, [Kk]
  Add4/1 -> MatrixMultiply7/1
  MatrixMultiply4/1 -> Add2/2
  [Kk] -> MatrixMultiply4/1
  [Z] -> Add3/1
  MatrixMultiply10/1 -> MatrixMultiply5/1, LDL Solver1/2
  MatrixMultiply5/1 -> Add5/1
  LDL Solver1/1 -> Math Function6/1
  [H] -> Math Function5/1
  [Pk_k_1] -> MatrixMultiply10/2
  [R] -> Add5/2
  Constant/1 -> Add4/1
  [Kk] -> MatrixMultiply6/1
  [Xk_k_1] -> Add2/1
  [H] -> MatrixMultiply6/2
  [H] -> MatrixMultiply9/1
  [Xk_k_1] -> MatrixMultiply9/2
  [Pk_k_1] -> MatrixMultiply7/2
  R/1 -> [R]
  Add5/1 -> LDL Solver1/1
  MatrixMultiply6/1 -> Add4/2
  H/1 -> [H]
  Add2/1 -> XOut/1
  Xkk/1 -> [Xk_k_1]
  Z/1 -> [Z]
  Pkk/1 -> [Pk_k_1]

== matlab function NavV1_0421_2021a/Sensor_Data_Process/Magn_Data_Process/gyro_preprocessing/MATLAB Function3 ==
  data: curr_input input single; curr_output output single; sample_freq input single; cutoff_freq input single
function curr_output = second_LPF_Butter_x(curr_input,sample_freq,cutoff_freq)
   persistent input_x;
   persistent output_x;

   if isempty(input_x)
       input_x = [0;0;0];
   end
   
   if isempty(output_x)
       output_x = [0;0;0];
   end
    B = [0,0,0];
    A = [0,0,0];
    M_PI_F = 3.1415926;
	fr = sample_freq / cutoff_freq;
	ohm = tan( M_PI_F / fr );
	c = 1.0 + 2.0 * cos( M_PI_F / 4.0 ) * ohm + ohm * ohm;
	B(1) = ohm * ohm / c;
	B(2) = 2.0 * B(1);
	B(3) = B(1);
	A(1) = 2.0 * ( ohm * ohm - 1.0) / c;
	A(2) = (1.0 - 2.0 * cos( M_PI_F / 4.0 ) * ohm + ohm * ohm) / c;
	%/*获取最新输入*/
	input_x(3) = curr_input;
	%/* Butterworth */
	output_x(3) =B(1) * input_x(3) + B(2) * input_x(2) +B(3) * input_x(1) - A(1) * output_x(2) - A(2) * output_x(1);
	curr_output =single(output_x(3));
   % /* 输入序列保存 */
	input_x(1) = input_x(2);
	input_x(2) = input_x(3);
	%/*输出序列保存 */
	output_x(1) = output_x(2);
	output_x(2) = output_x(3);

== matlab function NavV1_0421_2021a/Sensor_Data_Process/TOF_Data_Process/TD_baro/MATLAB Function2 ==
  data: T input single; u1 output; u0 input; u1 input single; u2 input single; h input single; r input single; u2 output
function [u1,u2]=diff_TD_2(T,u0,u1,u2,h,r)
    %init
    %T是信号周期，u0原始信号输入，u1跟踪原始信号，u2原始信号差分值，
    %h滤波因子（h=T时接近一阶差分）越大滤波好延迟大；r速度因子，越大跟踪的越快但是噪声放大；

	x1=0, x2=0;
	delta=0;
	delta0=0;
	y=0;
	fabs_y=0;
	a0=0;
	a=0;
    fst=0;
    
	x1 = u1;
	x2 = u2;
	delta = r*h;
	delta0 = delta*h;
	y = x1 - u0 + h*x2;
	fabs_y = abs(y);   
	a0 = sqrt(delta*delta + 8 * r*fabs_y);
    
	if (fabs_y <= delta0)
		a = x2 + y / h;
    else
        a = x2 + 0.5*(a0 - delta)*sign(y);
    end
    
	if (abs(a) <= delta)
		fst = -r*a / delta;
    else
		fst = -r*sign(a);
    end
	u1 = single(x1 + T*x2); %计算跟踪信号
	u2 = single(x2 + T*fst); % 计算微分信号

== matlab function NavV1_0421_2021a/State estimation/AHRS/att_update/QuatMult ==
  data: quatA input; quatOut output single; quatB input
function quatOut = QuatMult(quatA,quatB)
% Calculate the following quaternion product quatA * quatB using the 
% standard identity 

quatOut = [quatA(1)*quatB(1)-quatA(2:4)'*quatB(2:4); quatA(1)*quatB(2:4) + quatB(1)*quatA(2:4) + cross(quatA(2:4),quatB(2:4))];

== matlab function NavV1_0421_2021a/Sensor_Data_Process/IMU_Data_Process/accl_preprocessing/MATLAB Function1 ==
  data: curr_input input; curr_output output single; sample_freq input; cutoff_freq input
function curr_output = second_LPF_Butter_x(curr_input,sample_freq,cutoff_freq)
   persistent input_x;
   persistent output_x;

   if isempty(input_x)
       input_x = [0;0;0];
   end
   
   if isempty(output_x)
       output_x = [0;0;0];
   end
    B = [0,0,0];
    A = [0,0,0];
    M_PI_F = 3.1415926;
	fr = sample_freq / cutoff_freq;
	ohm = tan( M_PI_F / fr );
	c = 1.0 + 2.0 * cos( M_PI_F / 4.0 ) * ohm + ohm * ohm;
	B(1) = ohm * ohm / c;
	B(2) = 2.0 * B(1);
	B(3) = B(1);
	A(1) = 2.0 * ( ohm * ohm - 1.0) / c;
	A(2) = (1.0 - 2.0 * cos( M_PI_F / 4.0 ) * ohm + ohm * ohm) / c;
	%/*获取最新输入*/
	input_x(3) = curr_input;
	%/* Butterworth */
	output_x(3) =B(1) * input_x(3) + B(2) * input_x(2) +B(3) * input_x(1) - A(1) * output_x(2) - A(2) * output_x(1);
	curr_output = single(output_x(3));
   % /* 输入序列保存 */
	input_x(1) = input_x(2);
	input_x(2) = input_x(3);
	%/*输出序列保存 */
	output_x(1) = output_x(2);
	output_x(2) = output_x(3);

== matlab function NavV1_0421_2021a/State estimation/AHRS/att_update/rv2q ==
  data: rotVec input single; quaternion output single
% convert froma rotation vector in radians to a quaternion
function quaternion = RotToQuat(rotVec)

vecLength = sqrt(rotVec(1)^2 + rotVec(2)^2 + rotVec(3)^2);

if vecLength < 1e-6
  quaternion = single([1;0;0;0]);
else
  quaternion = single([cos(0.5*vecLength); rotVec/vecLength*sin(0.5*vecLength)]);
end

== matlab function NavV1_0421_2021a/State estimation/AHRS/AHRS Complementary filter/Trace differentiator/MATLAB Function2 ==
  data: T input single; u1 output; u0 input single; u1 input single; u2 input single; h input single; r input single; u2 output
function [u1,u2]=diff_TD_2(T,u0,u1,u2,h,r)
    %init
    %T是信号周期，u0原始信号输入，u1跟踪原始信号，u2原始信号差分值，
    %h滤波因子（h=T时接近一阶差分）越大滤波好延迟大；r速度因子，越大跟踪的越快但是噪声放大；

	x1=0, x2=0;
	delta=0;
	delta0=0;
	y=0;
	fabs_y=0;
	a0=0;
	a=0;
    fst=0;
    
	x1 = u1;
	x2 = u2;
	delta = r*h;
	delta0 = delta*h;
	y = x1 - u0 + h*x2;
	fabs_y = abs(y);   
	a0 = sqrt(delta*delta + 8 * r*fabs_y);
	if (fabs_y <= delta0)
		a = x2 + y / h;
    else
		a = x2 + 0.5*(a0 - delta)*sign(y);
    end
    
	if (abs(a) <= delta)
		fst = -r*a / delta;
    else
		fst = -r*sign(a);
    end
	u1 = single(x1 + T*x2); %计算跟踪信号
	u2 = single(x2 + T*fst); % 计算微分信号

== matlab function NavV1_0421_2021a/State estimation/AHRS/AHRS Complementary filter/Trace differentiator/MATLAB Function3 ==
  data: T input single; u1 output; u0 input single; u1 input single; u2 input single; h input single; r input single; u2 output
function [u1,u2]=diff_TD_2(T,u0,u1,u2,h,r)
    %init
	x1=0, x2=0;
	delta=0;
	delta0=0;
	y=0;
	fabs_y=0;
	a0=0;
	a=0;
    fst=0;
    
	x1 = u1;
	x2 = u2;
	delta = r*h;
	delta0 = delta*h;
	y = x1 - u0 + h*x2;
	fabs_y = abs(y);   
	a0 = sqrt(delta*delta + 8 * r*fabs_y);
	if (fabs_y <= delta0)
		a = x2 + y / h;
    else
		a = x2 + 0.5*(a0 - delta)*sign(y);
    end
    
	if (abs(a) <= delta)
		fst = -r*a / delta;
    else
		fst = -r*sign(a);
    end
	u1 = single(x1 + T*x2); %计算跟踪信号
	u2 = single(x2 + T*fst); % 计算微分信号

== matlab function NavV1_0421_2021a/Sensor_Data_Process/IMU_Data_Process/gyro_preprocessing/MATLAB Function1 ==
  data: curr_input input single; curr_output output single; sample_freq input single; cutoff_freq input single
function curr_output = second_LPF_Butter_x(curr_input,sample_freq,cutoff_freq)
   persistent input_x;
   persistent output_x;

   if isempty(input_x)
       input_x = [0;0;0];
   end
   
   if isempty(output_x)
       output_x = [0;0;0];
   end
    B = [0,0,0];
    A = [0,0,0];
    M_PI_F = 3.1415926;
	fr = sample_freq / cutoff_freq;
	ohm = tan( M_PI_F / fr );
	c = 1.0 + 2.0 * cos( M_PI_F / 4.0 ) * ohm + ohm * ohm;
	B(1) = ohm * ohm / c;
	B(2) = 2.0 * B(1);
	B(3) = B(1);
	A(1) = 2.0 * ( ohm * ohm - 1.0) / c;
	A(2) = (1.0 - 2.0 * cos( M_PI_F / 4.0 ) * ohm + ohm * ohm) / c;
	%/*获取最新输入*/
	input_x(3) = curr_input;
	%/* Butterworth */
	output_x(3) =B(1) * input_x(3) + B(2) * input_x(2) +B(3) * input_x(1) - A(1) * output_x(2) - A(2) * output_x(1);
	curr_output = single(output_x(3));
   % /* 输入序列保存 */
	input_x(1) = input_x(2);
	input_x(2) = input_x(3);
	%/*输出序列保存 */
	output_x(1) = output_x(2);
	output_x(2) = output_x(3);

== matlab function NavV1_0421_2021a/Sensor_Data_Process/IMU_Data_Process/gyro_preprocessing/MATLAB Function2 ==
  data: curr_input input single; curr_output output single; sample_freq input single; cutoff_freq input single
function curr_output = second_LPF_Butter_x(curr_input,sample_freq,cutoff_freq)
   persistent input_x;
   persistent output_x;

   if isempty(input_x)
       input_x = [0;0;0];
   end
   
   if isempty(output_x)
       output_x = [0;0;0];
   end
    B = [0,0,0];
    A = [0,0,0];
    M_PI_F = 3.1415926;
	fr = sample_freq / cutoff_freq;
	ohm = tan( M_PI_F / fr );
	c = 1.0 + 2.0 * cos( M_PI_F / 4.0 ) * ohm + ohm * ohm;
	B(1) = ohm * ohm / c;
	B(2) = 2.0 * B(1);
	B(3) = B(1);
	A(1) = 2.0 * ( ohm * ohm - 1.0) / c;
	A(2) = (1.0 - 2.0 * cos( M_PI_F / 4.0 ) * ohm + ohm * ohm) / c;
	%/*获取最新输入*/
	input_x(3) = curr_input;
	%/* Butterworth */
	output_x(3) =B(1) * input_x(3) + B(2) * input_x(2) +B(3) * input_x(1) - A(1) * output_x(2) - A(2) * output_x(1);
	curr_output = single(output_x(3));
   % /* 输入序列保存 */
	input_x(1) = input_x(2);
	input_x(2) = input_x(3);
	%/*输出序列保存 */
	output_x(1) = output_x(2);
	output_x(2) = output_x(3);

== matlab function NavV1_0421_2021a/Sensor_Data_Process/IMU_Data_Process/gyro_preprocessing/MATLAB Function3 ==
  data: curr_input input single; curr_output output single; sample_freq input single; cutoff_freq input single
function curr_output = second_LPF_Butter_x(curr_input,sample_freq,cutoff_freq)
   persistent input_x;
   persistent output_x;

   if isempty(input_x)
       input_x = [0;0;0];
   end
   
   if isempty(output_x)
       output_x = [0;0;0];
   end
    B = [0,0,0];
    A = [0,0,0];
    M_PI_F = 3.1415926;
	fr = sample_freq / cutoff_freq;
	ohm = tan( M_PI_F / fr );
	c = 1.0 + 2.0 * cos( M_PI_F / 4.0 ) * ohm + ohm * ohm;
	B(1) = ohm * ohm / c;
	B(2) = 2.0 * B(1);
	B(3) = B(1);
	A(1) = 2.0 * ( ohm * ohm - 1.0) / c;
	A(2) = (1.0 - 2.0 * cos( M_PI_F / 4.0 ) * ohm + ohm * ohm) / c;
	%/*获取最新输入*/
	input_x(3) = curr_input;
	%/* Butterworth */
	output_x(3) =B(1) * input_x(3) + B(2) * input_x(2) +B(3) * input_x(1) - A(1) * output_x(2) - A(2) * output_x(1);
	curr_output = single(output_x(3));
   % /* 输入序列保存 */
	input_x(1) = input_x(2);
	input_x(2) = input_x(3);
	%/*输出序列保存 */
	output_x(1) = output_x(2);
	output_x(2) = output_x(3);

== matlab function NavV1_0421_2021a/Sensor_Data_Process/IMU_Data_Process/accl_preprocessing/MATLAB Function2 ==
  data: curr_input input; curr_output output single; sample_freq input; cutoff_freq input
function curr_output = second_LPF_Butter_x(curr_input,sample_freq,cutoff_freq)
   persistent input_x;
   persistent output_x;

   if isempty(input_x)
       input_x = [0;0;0];
   end
   
   if isempty(output_x)
       output_x = [0;0;0];
   end
    B = [0,0,0];
    A = [0,0,0];
    M_PI_F = 3.1415926;
	fr = sample_freq / cutoff_freq;
	ohm = tan( M_PI_F / fr );
	c = 1.0 + 2.0 * cos( M_PI_F / 4.0 ) * ohm + ohm * ohm;
	B(1) = ohm * ohm / c;
	B(2) = 2.0 * B(1);
	B(3) = B(1);
	A(1) = 2.0 * ( ohm * ohm - 1.0) / c;
	A(2) = (1.0 - 2.0 * cos( M_PI_F / 4.0 ) * ohm + ohm * ohm) / c;
	%/*获取最新输入*/
	input_x(3) = curr_input;
	%/* Butterworth */
	output_x(3) =B(1) * input_x(3) + B(2) * input_x(2) +B(3) * input_x(1) - A(1) * output_x(2) - A(2) * output_x(1);
	curr_output = single(output_x(3));
   % /* 输入序列保存 */
	input_x(1) = input_x(2);
	input_x(2) = input_x(3);
	%/*输出序列保存 */
	output_x(1) = output_x(2);
	output_x(2) = output_x(3);

== matlab function NavV1_0421_2021a/Sensor_Data_Process/IMU_Data_Process/accl_preprocessing/MATLAB Function3 ==
  data: curr_input input; curr_output output single; sample_freq input; cutoff_freq input
function curr_output = second_LPF_Butter_x(curr_input,sample_freq,cutoff_freq)
   persistent input_x;
   persistent output_x;

   if isempty(input_x)
       input_x = [0;0;0];
   end
   
   if isempty(output_x)
       output_x = [0;0;0];
   end
    B = [0,0,0];
    A = [0,0,0];
    M_PI_F = 3.1415926;
	fr = sample_freq / cutoff_freq;
	ohm = tan( M_PI_F / fr );
	c = 1.0 + 2.0 * cos( M_PI_F / 4.0 ) * ohm + ohm * ohm;
	B(1) = ohm * ohm / c;
	B(2) = 2.0 * B(1);
	B(3) = B(1);
	A(1) = 2.0 * ( ohm * ohm - 1.0) / c;
	A(2) = (1.0 - 2.0 * cos( M_PI_F / 4.0 ) * ohm + ohm * ohm) / c;
	%/*获取最新输入*/
	input_x(3) = curr_input;
	%/* Butterworth */
	output_x(3) =B(1) * input_x(3) + B(2) * input_x(2) +B(3) * input_x(1) - A(1) * output_x(2) - A(2) * output_x(1);
	curr_output = single(output_x(3));
   % /* 输入序列保存 */
	input_x(1) = input_x(2);
	input_x(2) = input_x(3);
	%/*输出序列保存 */
	output_x(1) = output_x(2);
	output_x(2) = output_x(3);

== matlab function NavV1_0421_2021a/Sensor_Data_Process/baro_Data_Process/TD_baro/MATLAB Function2 ==
  data: T input single; u1 output; u0 input; u1 input single; u2 input single; h input single; r input single; u2 output
function [u1,u2]=diff_TD_2(T,u0,u1,u2,h,r)
    %init
    %T是信号周期，u0原始信号输入，u1跟踪原始信号，u2原始信号差分值，
    %h滤波因子（h=T时接近一阶差分）越大滤波好延迟大；r速度因子，越大跟踪的越快但是噪声放大；

	x1=0, x2=0;
	delta=0;
	delta0=0;
	y=0;
	fabs_y=0;
	a0=0;
	a=0;
    fst=0;
    
	x1 = u1;
	x2 = u2;
	delta = r*h;
	delta0 = delta*h;
	y = x1 - u0 + h*x2;
	fabs_y = abs(y);   
	a0 = sqrt(delta*delta + 8 * r*fabs_y);
    
	if (fabs_y <= delta0)
		a = x2 + y / h;
    else
        a = x2 + 0.5*(a0 - delta)*sign(y);
    end
    
	if (abs(a) <= delta)
		fst = -r*a / delta;
    else
		fst = -r*sign(a);
    end
	u1 = single(x1 + T*x2); %计算跟踪信号
	u2 = single(x2 + T*fst); % 计算微分信号

== matlab function NavV1_0421_2021a/State estimation/AHRS/AHRS Complementary filter/manoeuvrable check/manoeuvrable check/manoeuvrable check ==
  data: flag output; fn input
function flag = fcn(fn)
    if abs(fn(1)) <0.8 && abs(fn(2))<0.8 && abs(fn(3)-9.79)<0.5
        flag = 1;
    else
        flag = 0;
    end
end

== matlab function NavV1_0421_2021a/State estimation/AHRS/AHRS Complementary filter/Trace differentiator/MATLAB Function1 ==
  data: T input single; u1 output; u0 input single; u1 input single; u2 input single; h input single; r input single; u2 output
function [u1,u2]=diff_TD_2(T,u0,u1,u2,h,r)
    %init
	x1=0, x2=0;
	delta=0;
	delta0=0;
	y=0;
	fabs_y=0;
	a0=0;
	a=0;
    fst=0;
    
	x1 = u1;
	x2 = u2;
	delta = r*h;
	delta0 = delta*h;
	y = x1 - u0 + h*x2;
	fabs_y = abs(y);   
	a0 = sqrt(delta*delta + 8 * r*fabs_y);
	if (fabs_y <= delta0)
		a = x2 + y / h;
    else
		a = x2 + 0.5*(a0 - delta)*sign(y);
    end
    
	if (abs(a) <= delta)
		fst = -r*a / delta;
    else
		fst = -r*sign(a);
    end
	u1 = x1 + T*x2; %计算跟踪信号
	u2 = x2 + T*fst; % 计算微分信号

== matlab function NavV1_0421_2021a/read IMUdata3/TD_baro/MATLAB Function2 ==
  data: T input single; u1 output; u0 input; u1 input single; u2 input single; h input single; r input single; u2 output
function [u1,u2]=diff_TD_2(T,u0,u1,u2,h,r)
    %init
    %T是信号周期，u0原始信号输入，u1跟踪原始信号，u2原始信号差分值，
    %h滤波因子（h=T时接近一阶差分）越大滤波好延迟大；r速度因子，越大跟踪的越快但是噪声放大；

	x1=0, x2=0;
	delta=0;
	delta0=0;
	y=0;
	fabs_y=0;
	a0=0;
	a=0;
    fst=0;
    
	x1 = u1;
	x2 = u2;
	delta = r*h;
	delta0 = delta*h;
	y = x1 - u0 + h*x2;
	fabs_y = abs(y);   
	a0 = sqrt(delta*delta + 8 * r*fabs_y);
    
	if (fabs_y <= delta0)
		a = x2 + y / h;
    else
        a = x2 + 0.5*(a0 - delta)*sign(y);
    end
    
	if (abs(a) <= delta)
		fst = -r*a / delta;
    else
		fst = -r*sign(a);
    end
	u1 = single(x1 + T*x2); %计算跟踪信号
	u2 = single(x2 + T*fst); % 计算微分信号

== matlab function NavV1_0421_2021a/Sensor_Data_Process/Magn_Data_Process/gyro_preprocessing/MATLAB Function1 ==
  data: curr_input input single; curr_output output single; sample_freq input single; cutoff_freq input single
function curr_output = second_LPF_Butter_x(curr_input,sample_freq,cutoff_freq)
   persistent input_x;
   persistent output_x;

   if isempty(input_x)
       input_x = [0;0;0];
   end
   
   if isempty(output_x)
       output_x = [0;0;0];
   end
    B = [0,0,0];
    A = [0,0,0];
    M_PI_F = 3.1415926;
	fr = sample_freq / cutoff_freq;
	ohm = tan( M_PI_F / fr );
	c = 1.0 + 2.0 * cos( M_PI_F / 4.0 ) * ohm + ohm * ohm;
	B(1) = ohm * ohm / c;
	B(2) = 2.0 * B(1);
	B(3) = B(1);
	A(1) = 2.0 * ( ohm * ohm - 1.0) / c;
	A(2) = (1.0 - 2.0 * cos( M_PI_F / 4.0 ) * ohm + ohm * ohm) / c;
	%/*获取最新输入*/
	input_x(3) = curr_input;
	%/* Butterworth */
	output_x(3) =B(1) * input_x(3) + B(2) * input_x(2) +B(3) * input_x(1) - A(1) * output_x(2) - A(2) * output_x(1);
	curr_output = single(output_x(3));
   % /* 输入序列保存 */
	input_x(1) = input_x(2);
	input_x(2) = input_x(3);
	%/*输出序列保存 */
	output_x(1) = output_x(2);
	output_x(2) = output_x(3);
